simulink model "Mainframe"  (R2021a)
settings: Solver=FixedStepAuto  StartTime=0.0  StopTime=60  FixedStep=0.001  RelTol=1e-3
values from neighbouring files (symbols this model uses):
  den_lpf_d = den_lpf20    [Mainframe_init.m]    (also in load_autopilot.m)
  Emulated_FCC_IO_Delay = 7    [Mainframe_init.m]
  Enable_Gyros = 0    [Mainframe_init.m]
  Enable_INS = 0    [Mainframe_init.m]
  num_lpf_d = num_lpf20    [Mainframe_init.m]    (also in load_autopilot.m)
undefined symbols (not defined in the file or in its folder): act_dmp, act_omega, Actuator, Aerodynamics, aMode, Autopilot, AUX, c_b_WGS, c_be, c_flat, c_grav, c_h_geop0, c_h_geope, c_pa0, c_pe, c_r0, c_rot, c_rsma, c_Tmp0, d_siB_0, d_siB_max, d_siB_min, dd_siB_max, dd_siB_min, dev, DiscIntNeverNeededParam, e_pa, e_Tmp, fin_maxrate, flag_I_act_switch, flag_I_aero_switch, flag_I_flat, flag_I_gravity_switch, flag_I_rot, hcr, HIL_Data, JMMM_0, JMMM_e, JSPB_e, lat_0, lon_0, Mass_Props, mB_0, mM_0, mM_e, National_Instruments, Newton, pBII_0, PCIe, pMPB, pNPB, propellant_kg, prp_FBPB, prp_mdot, prp_T, pSPB, pwm_output1, qEG_0, qIB_0, qIE_0 ... (+31)
libraries: simulink_extras x38, simulink x31, custom_blocks x11, sldrtlib x10, aerolibcommonsys x4, px4Sensorslib x3, px4lib x3, aerolibnav x1
(part 13 of 17)

== system Mainframe/Non-linear Flight Dynamic Model/GRM_Airframe/rb_eom/eom_6dof/Rigid_Body_EOM_6_DOF/rb_eom_6dof/calc_d_qIB ==
  note: Body-Drehraten
      | d_qBI(1) =1/2 { q4wx  - q3wy + q2wz }
      | d_qBI(2) =1/2 { q3wx + q4wy  - q1wz }
      | d_qBI(3) =1/2 {-q2wx + q1wy + q4wz }
      | d_qBI(4) =1/2 {-q1wx  - q2wy  - q3wz }
      |
      | Entspricht Zipfel (s. 372, Gl 10.11)
      | Entspricht "Representing Attitude: Euler angles, Unit Quaternions, and Rotation Vectors",
      | 	J. Diebel, Stanford University, S. 16, Gl 157 oder (159 & 151)
      |
      | d_qBI = 1/2 * [wBIB (1, 2, 3), 0] * qBI
  qIB : Inport
  wBIB : Inport  Port=2
  Add : Sum  Inputs=++++
  Constant : Constant  Value=0
  Demux : Demux  Outputs=3
  Demux1 : Demux
  Gain : Gain  Gain=0.5
  Product{2..5} (4 alike) : Product
  Product6 : Product  Multiplication=Matrix(*)
  Q_1 : Constant  Value=[0 0 0 1; 0 0 1 0; 0 -1 0 0; -1 0 0 0]
  Q_2 : Constant  Value=[0 0 -1 0; 0 0 0 1; 1 0 0 0; 0 -1 0 0]
  Q_3 : Constant  Value=[0 1 0 0; -1 0 0 0; 0 0 0 1; 0 0 -1 0]
  Q_4 : Constant  Value=[1 0 0 0; 0 1 0 0; 0 0 1 0; 0 0 0 1]
  Vector Concatenate : Concatenate  NumInputs=4
  conjugate_quaternion : Subsystem
      mask help: conjugate a quaternion
      mask Help:
      | Name:
      | 
      |     conjugate_quaternion
      | 
      | Description:
      | 
      |     computes the conjugate quaternion
      | 
      | Inputs  [size] [data type] [unit]:
      | 
      |     quaternion q_2_1  [4] [double] [-]
      | 
      | Outputs  [size] [data type] [unit]:
      | 
      |     conjugated quaternion q_1_2  [4] [double] [-]
      mask Display: disp (' conj(q)')
  conjugate_quaternion1 : Subsystem
      mask help: conjugate a quaternion
      mask Help:
      | Name:
      | 
      |     conjugate_quaternion
      | 
      | Description:
      | 
      |     computes the conjugate quaternion
      | 
      | Inputs  [size] [data type] [unit]:
      | 
      |     quaternion q_2_1  [4] [double] [-]
      | 
      | Outputs  [size] [data type] [unit]:
      | 
      |     conjugated quaternion q_1_2  [4] [double] [-]
      mask Display: disp (' conj(q)')
  d_qIB : Outport  VectorParamsAs1DForOutWhenUnconnected=off
  wires:
  conjugate_quaternion1/1(q_conj) -> d_qIB/1  "d_qIB"
  conjugate_quaternion/1(q_conj) -> Product6/2  "qBI"
  Vector Concatenate/1 -> Demux1/1
  Constant/1 -> Vector Concatenate/4
  Demux/3 -> Vector Concatenate/3
  Demux/2 -> Vector Concatenate/2
  Demux/1 -> Vector Concatenate/1
  wBIB/1 -> Demux/1
  qIB/1 -> conjugate_quaternion/1(q)
  Gain/1 -> conjugate_quaternion1/1(q)  "d_qBI"
  Product2/1 -> Add/1
  Product4/1 -> Add/3
  Demux1/4 -> Product5/2  "w4"
  Demux1/3 -> Product4/2  "w3"
  Product3/1 -> Add/2
  Q_2/1 -> Product3/1
  Q_1/1 -> Product2/1
  Demux1/2 -> Product3/2  "w2"
  Q_4/1 -> Product5/1
  Product6/1 -> Gain/1
  Product5/1 -> Add/4
  Demux1/1 -> Product2/2  "w1"
  Add/1 -> Product6/1  "Q(w')"
  Q_3/1 -> Product4/1

== system Mainframe/Non-linear Flight Dynamic Model/GRM_Airframe/rb_eom/eom_6dof/Rigid_Body_EOM_6_DOF/rb_eom_6dof/cross_product ==
  note: Outputs [size]:
      |
      | r1 x r2  [3x1]
  note: Inputs [size]:
      |
      | r1 [3x1]
      | r2 [3x1]
  r1 : Inport
  r2 : Inport  Port=2
  Demux2 : Demux  Outputs=[1;1;1]
      settings: DisplayOption=none
  Demux3 : Demux  Outputs=[1;1;1]
      settings: DisplayOption=none
  Product{2..7} (6 alike) : Product  InputSameDT=on  RndMeth=Zero  SaturateOnIntegerOverflow=on  OutDataTypeStr=Inherit: Same as first input
  Sum : Sum  Inputs=+-  InputSameDT=on  SaturateOnIntegerOverflow=on  OutDataTypeStr=Inherit: Same as first input
  Sum1 : Sum  Inputs=+-  InputSameDT=on  SaturateOnIntegerOverflow=on  OutDataTypeStr=Inherit: Same as first input
  Sum2 : Sum  Inputs=+-  InputSameDT=on  SaturateOnIntegerOverflow=on  OutDataTypeStr=Inherit: Same as first input
  Vector Concatenate : Concatenate  NumInputs=3  Mode=Multidimensional array
  r1_x_r2 : Outport  PortDimensions=[3,1]  VectorParamsAs1DForOutWhenUnconnected=off
  wires:
  Demux2/2 -> Product2/1, Product7/1
  Demux3/3 -> Product5/2, Product2/2
  Demux3/2 -> Product6/2, Product3/2
  Demux2/3 -> Product3/1, Product4/1
  Demux3/1 -> Product7/2, Product4/2
  Demux2/1 -> Product6/1, Product5/1
  Product2/1 -> Sum/1
  Product3/1 -> Sum/2
  Product4/1 -> Sum1/1
  Product5/1 -> Sum1/2
  Product6/1 -> Sum2/1
  Product7/1 -> Sum2/2
  Sum/1 -> Vector Concatenate/1
  Sum1/1 -> Vector Concatenate/2
  Sum2/1 -> Vector Concatenate/3
  r1/1 -> Demux2/1
  r2/1 -> Demux3/1
  Vector Concatenate/1 -> r1_x_r2/1

== system Mainframe/Non-linear Flight Dynamic Model/GRM_Airframe/rb_eom/eom_6dof/Rigid_Body_EOM_6_DOF/rb_eom_6dof/r2_from_r1_trans_q21 ==
  note: Outputs [size]:
      |
      | vector r2 [3]
  note: Inputs [size]:
      |
      | vector r1 [3]
      | quaternion q21 [4]
  r1 : Inport
  q21 : Inport  Port=2
  Add : Sum  Inputs=++++
  Add1 : Sum  Inputs=++++
  Constant : Constant  Value=0
  Demux : Demux  Outputs=3
  Demux1 : Demux
  Demux2 : Demux
  Math Function : Math  Operator=transpose  SignedPower=on  SaturateOnIntegerOverflow=on
  Product{,1..7} (8 alike) : Product
  Product8 : Product  Inputs=3  Multiplication=Matrix(*)
  Q_1 : Constant  Value=[0 0 0 1; 0 0 1 0; 0 -1 0 0; -1 0 0 0]
  Q_2 : Constant  Value=[0 0 -1 0; 0 0 0 1; 1 0 0 0; 0 -1 0 0]
  Q_3 : Constant  Value=[0 1 0 0; -1 0 0 0; 0 0 0 1; 0 0 -1 0]
  Q_4 : Constant  Value=[1 0 0 0; 0 1 0 0; 0 0 1 0; 0 0 0 1]
  Q~_1 : Constant  Value=[0 0 0 1; 0 0 -1 0; 0 1 0 0; -1 0 0 0]
  Q~_2 : Constant  Value=[0 0 1 0; 0 0 0 1; -1 0 0 0; 0 -1 0 0]
  Q~_3 : Constant  Value=[0 -1 0 0; 1 0 0 0; 0 0 0 1; 0 0 -1 0]
  Q~_4 : Constant  Value=[1 0 0 0; 0 1 0 0; 0 0 1 0; 0 0 0 1]
  Selector : Selector  IndexMode=Zero-based  InputPortWidth=4  IndexOptions=Index vector (dialog)  Indices=[0 1 2]  OutputSizes=1
  Vector Concatenate : Concatenate  NumInputs=4
  r2 : Outport  VectorParamsAs1DForOutWhenUnconnected=off
  wires:
  Selector/1 -> r2/1
  Product8/1 -> Selector/1
  Vector Concatenate/1 -> Product8/3
  Constant/1 -> Vector Concatenate/4
  Math Function/1 -> Product8/1  "Q~T(q)"
  Q~_3/1 -> Product6/1
  Q~_1/1 -> Product4/1
  Q~_4/1 -> Product7/1
  Product6/1 -> Add1/3
  Demux2/3 -> Product6/2  "q3"
  Product5/1 -> Add1/2
  Demux2/2 -> Product5/2  "q2"
  Add1/1 -> Math Function/1  "Q~(q)"
  q21/1 -> Demux1/1, Demux2/1
  Product7/1 -> Add1/4
  Product4/1 -> Add1/1
  Q~_2/1 -> Product5/1
  Demux2/4 -> Product7/2  "q4"
  Demux2/1 -> Product4/2  "q1"
  Add/1 -> Product8/2  "Q(q)"
  Product3/1 -> Add/4
  Product2/1 -> Add/3
  Product1/1 -> Add/2
  Product/1 -> Add/1
  Q_4/1 -> Product3/1
  Q_3/1 -> Product2/1
  Q_2/1 -> Product1/1
  Q_1/1 -> Product/1
  Demux1/4 -> Product3/2  "q4"
  Demux1/3 -> Product2/2  "q3"
  Demux1/2 -> Product1/2  "q2"
  Demux1/1 -> Product/2  "q1"
  Demux/3 -> Vector Concatenate/3  "rz"
  Demux/2 -> Vector Concatenate/2  "ry"
  Demux/1 -> Vector Concatenate/1  "rx"
  r1/1 -> Demux/1

== system Mainframe/Non-linear Flight Dynamic Model/GRM_Airframe/stream_flow/calc_stream_flow/Subsystem1/AoA_Sideslip_Alphatot_Phi/norm_of_vector ==
  note: Outputs [size]:
      |
      | norm of vector [1]
  note: Inputs [size]:
      |
      | vector  [3]
  vector : Inport
  Dot Product1 : DotProduct  InputSameDT=on  OutDataTypeStr=Inherit: Inherit via internal rule
  Math Function1 : Math  Operator=sqrt  SignedPower=on  SaturateOnIntegerOverflow=on
  norm_of_vector : Outport  VectorParamsAs1DForOutWhenUnconnected=off
  wires:
  vector/1 -> Dot Product1/1, Dot Product1/2
  Math Function1/1 -> norm_of_vector/1
  Dot Product1/1 -> Math Function1/1

== system Mainframe/Non-linear Flight Dynamic Model/GRM_Airframe/weight_and_balance/moi/moi_coordinate_transformation/3_rot_mat/1. Rotation x-Achse ==
  alpha1 : Inport
  Constant : Constant
  Constant{1..2,7..8} (4 alike) : Constant  Value=0
  Gain : Gain  Gain=-1
  Matrix Concatenate : Concatenate  NumInputs=3  Mode=Multidimensional array  ConcatenateDimension=2
  Mux : Mux  Inputs=3
  Mux1 : Mux  Inputs=3
  Mux2 : Mux  Inputs=3
  Trigonometric Function : Trigonometry  Operator=cos
  Trigonometric Function1 : Trigonometry
  Trigonometric Function2 : Trigonometry
  Trigonometric Function3 : Trigonometry  Operator=cos
  1Rot_Matrix_x : Outport  VectorParamsAs1DForOutWhenUnconnected=off
  wires:
  Gain/1 -> Mux1/3
  alpha1/1 -> Trigonometric Function2/1, Trigonometric Function/1, Trigonometric Function1/1, Trigonometric Function3/1
  Constant/1 -> Mux/1
  Constant1/1 -> Mux/2
  Constant2/1 -> Mux/3
  Constant8/1 -> Mux1/1
  Trigonometric Function/1 -> Mux1/2
  Trigonometric Function2/1 -> Gain/1
  Constant7/1 -> Mux2/1
  Trigonometric Function1/1 -> Mux2/2
  Trigonometric Function3/1 -> Mux2/3
  Mux/1 -> Matrix Concatenate/1
  Mux1/1 -> Matrix Concatenate/2
  Mux2/1 -> Matrix Concatenate/3
  Matrix Concatenate/1 -> 1Rot_Matrix_x/1

== system Mainframe/Non-linear Flight Dynamic Model/GRM_Airframe/weight_and_balance/moi/moi_coordinate_transformation/3_rot_mat/1. Rotation y-Achse ==
  alpha1 : Inport
  Constant{,2,7..8} (4 alike) : Constant  Value=0
  Constant1 : Constant
  Gain1 : Gain  Gain=-1
  Matrix Concatenate : Concatenate  NumInputs=3  Mode=Multidimensional array  ConcatenateDimension=2
  Mux : Mux  Inputs=3
  Mux1 : Mux  Inputs=3
  Mux2 : Mux  Inputs=3
  Trigonometric Function : Trigonometry  Operator=cos
  Trigonometric Function1 : Trigonometry
  Trigonometric Function2 : Trigonometry
  Trigonometric Function3 : Trigonometry  Operator=cos
  1Rot_Matrix_y : Outport  VectorParamsAs1DForOutWhenUnconnected=off
  wires:
  Gain1/1 -> Mux2/1
  Mux2/1 -> Matrix Concatenate/3
  Mux1/1 -> Matrix Concatenate/2
  Mux/1 -> Matrix Concatenate/1
  Trigonometric Function3/1 -> Mux2/3
  Trigonometric Function1/1 -> Gain1/1
  Constant2/1 -> Mux1/3
  Constant1/1 -> Mux1/2
  Constant/1 -> Mux1/1
  alpha1/1 -> Trigonometric Function1/1, Trigonometric Function3/1, Trigonometric Function2/1, Trigonometric Function/1
  Constant8/1 -> Mux/2
  Trigonometric Function/1 -> Mux/1
  Trigonometric Function2/1 -> Mux/3
  Constant7/1 -> Mux2/2
  Matrix Concatenate/1 -> 1Rot_Matrix_y/1

== system Mainframe/Non-linear Flight Dynamic Model/GRM_Airframe/weight_and_balance/moi/moi_coordinate_transformation/3_rot_mat/1. Rotation z-Achse ==
  alpha1 : Inport
  Constant{4,7..8,10} (4 alike) : Constant  Value=0
  Constant11 : Constant
  Gain : Gain  Gain=-1
  Matrix Concatenate : Concatenate  NumInputs=3  Mode=Multidimensional array  ConcatenateDimension=2
  Mux : Mux  Inputs=3
  Mux1 : Mux  Inputs=3
  Mux2 : Mux  Inputs=3
  Trigonometric Function : Trigonometry  Operator=cos
  Trigonometric Function1 : Trigonometry
  Trigonometric Function3 : Trigonometry  Operator=cos
  Trigonometric Function4 : Trigonometry
  1Rot_Matrix_z : Outport  VectorParamsAs1DForOutWhenUnconnected=off
  wires:
  Gain/1 -> Mux/2
  Trigonometric Function/1 -> Mux1/2
  Mux/1 -> Matrix Concatenate/1
  Mux1/1 -> Matrix Concatenate/2
  Mux2/1 -> Matrix Concatenate/3
  Trigonometric Function1/1 -> Mux1/1
  Constant7/1 -> Mux1/3
  Constant4/1 -> Mux2/1
  Constant10/1 -> Mux2/2
  Constant11/1 -> Mux2/3
  Trigonometric Function3/1 -> Mux/1
  Trigonometric Function4/1 -> Gain/1
  Constant8/1 -> Mux/3
  Matrix Concatenate/1 -> 1Rot_Matrix_z/1
  alpha1/1 -> Trigonometric Function3/1, Trigonometric Function4/1, Trigonometric Function/1, Trigonometric Function1/1

== system Mainframe/Non-linear Flight Dynamic Model/GRM_Airframe/weight_and_balance/moi/moi_coordinate_transformation/3_rot_mat/2. Rotation x-Achse ==
  alpha2 : Inport
  Constant : Constant
  Constant{1..2,7..8} (4 alike) : Constant  Value=0
  Gain : Gain  Gain=-1
  Matrix Concatenate : Concatenate  NumInputs=3  Mode=Multidimensional array  ConcatenateDimension=2
  Mux : Mux  Inputs=3
  Mux1 : Mux  Inputs=3
  Mux2 : Mux  Inputs=3
  Trigonometric Function : Trigonometry  Operator=cos
  Trigonometric Function1 : Trigonometry
  Trigonometric Function2 : Trigonometry
  Trigonometric Function3 : Trigonometry  Operator=cos
  2Rot_Matrix_x : Outport  VectorParamsAs1DForOutWhenUnconnected=off
  wires:
  Gain/1 -> Mux1/3
  alpha2/1 -> Trigonometric Function2/1, Trigonometric Function/1, Trigonometric Function1/1, Trigonometric Function3/1
  Constant/1 -> Mux/1
  Constant1/1 -> Mux/2
  Constant2/1 -> Mux/3
  Constant8/1 -> Mux1/1
  Trigonometric Function/1 -> Mux1/2
  Trigonometric Function2/1 -> Gain/1
  Constant7/1 -> Mux2/1
  Trigonometric Function1/1 -> Mux2/2
  Trigonometric Function3/1 -> Mux2/3
  Mux/1 -> Matrix Concatenate/1
  Mux1/1 -> Matrix Concatenate/2
  Mux2/1 -> Matrix Concatenate/3
  Matrix Concatenate/1 -> 2Rot_Matrix_x/1

== system Mainframe/Non-linear Flight Dynamic Model/GRM_Airframe/weight_and_balance/moi/moi_coordinate_transformation/3_rot_mat/2. Rotation y-Achse ==
  alpha2 : Inport
  Constant{,2,7..8} (4 alike) : Constant  Value=0
  Constant1 : Constant
  Gain1 : Gain  Gain=-1
  Matrix Concatenate : Concatenate  NumInputs=3  Mode=Multidimensional array  ConcatenateDimension=2
  Mux : Mux  Inputs=3
  Mux1 : Mux  Inputs=3
  Mux2 : Mux  Inputs=3
  Trigonometric Function : Trigonometry  Operator=cos
  Trigonometric Function1 : Trigonometry
  Trigonometric Function2 : Trigonometry
  Trigonometric Function3 : Trigonometry  Operator=cos
  2Rot_Matrix_y : Outport  VectorParamsAs1DForOutWhenUnconnected=off
  wires:
  Gain1/1 -> Mux2/1
  Mux2/1 -> Matrix Concatenate/3
  Mux1/1 -> Matrix Concatenate/2
  Mux/1 -> Matrix Concatenate/1
  Trigonometric Function3/1 -> Mux2/3
  Trigonometric Function1/1 -> Gain1/1
  Constant2/1 -> Mux1/3
  Constant1/1 -> Mux1/2
  Constant/1 -> Mux1/1
  alpha2/1 -> Trigonometric Function1/1, Trigonometric Function3/1, Trigonometric Function2/1, Trigonometric Function/1
  Constant8/1 -> Mux/2
  Trigonometric Function/1 -> Mux/1
  Trigonometric Function2/1 -> Mux/3
  Constant7/1 -> Mux2/2
  Matrix Concatenate/1 -> 2Rot_Matrix_y/1

== system Mainframe/Non-linear Flight Dynamic Model/GRM_Airframe/weight_and_balance/moi/moi_coordinate_transformation/3_rot_mat/2. Rotation z-Achse ==
  alpha2 : Inport
  Constant{4,7..8,10} (4 alike) : Constant  Value=0
  Constant11 : Constant
  Gain : Gain  Gain=-1
  Matrix Concatenate : Concatenate  NumInputs=3  Mode=Multidimensional array  ConcatenateDimension=2
  Mux : Mux  Inputs=3
  Mux1 : Mux  Inputs=3
  Mux2 : Mux  Inputs=3
  Trigonometric Function : Trigonometry  Operator=cos
  Trigonometric Function1 : Trigonometry
  Trigonometric Function3 : Trigonometry  Operator=cos
  Trigonometric Function4 : Trigonometry
  2Rot_Matrix_z : Outport  VectorParamsAs1DForOutWhenUnconnected=off
  wires:
  Gain/1 -> Mux/2
  Trigonometric Function/1 -> Mux1/2
  Mux/1 -> Matrix Concatenate/1
  Mux1/1 -> Matrix Concatenate/2
  Mux2/1 -> Matrix Concatenate/3
  Trigonometric Function1/1 -> Mux1/1
  Constant7/1 -> Mux1/3
  Constant4/1 -> Mux2/1
  Constant10/1 -> Mux2/2
  Constant11/1 -> Mux2/3
  Trigonometric Function3/1 -> Mux/1
  Trigonometric Function4/1 -> Gain/1
  Constant8/1 -> Mux/3
  Matrix Concatenate/1 -> 2Rot_Matrix_z/1
  alpha2/1 -> Trigonometric Function3/1, Trigonometric Function4/1, Trigonometric Function/1, Trigonometric Function1/1

== system Mainframe/Non-linear Flight Dynamic Model/GRM_Airframe/weight_and_balance/moi/moi_coordinate_transformation/3_rot_mat/3. Rotation x-Achse ==
  alpha3 : Inport
  Constant : Constant
  Constant{1..2,7..8} (4 alike) : Constant  Value=0
  Gain : Gain  Gain=-1
  Matrix Concatenate : Concatenate  NumInputs=3  Mode=Multidimensional array  ConcatenateDimension=2
  Mux : Mux  Inputs=3
  Mux1 : Mux  Inputs=3
  Mux2 : Mux  Inputs=3
  Trigonometric Function : Trigonometry  Operator=cos
  Trigonometric Function1 : Trigonometry
  Trigonometric Function2 : Trigonometry
  Trigonometric Function3 : Trigonometry  Operator=cos
  3Rot_Matrix_x : Outport  VectorParamsAs1DForOutWhenUnconnected=off
  wires:
  Gain/1 -> Mux1/3
  alpha3/1 -> Trigonometric Function2/1, Trigonometric Function/1, Trigonometric Function1/1, Trigonometric Function3/1
  Constant/1 -> Mux/1
  Constant1/1 -> Mux/2
  Constant2/1 -> Mux/3
  Constant8/1 -> Mux1/1
  Trigonometric Function/1 -> Mux1/2
  Trigonometric Function2/1 -> Gain/1
  Constant7/1 -> Mux2/1
  Trigonometric Function1/1 -> Mux2/2
  Trigonometric Function3/1 -> Mux2/3
  Mux/1 -> Matrix Concatenate/1
  Mux1/1 -> Matrix Concatenate/2
  Mux2/1 -> Matrix Concatenate/3
  Matrix Concatenate/1 -> 3Rot_Matrix_x/1

== system Mainframe/Non-linear Flight Dynamic Model/GRM_Airframe/weight_and_balance/moi/moi_coordinate_transformation/3_rot_mat/3. Rotation y-Achse ==
  alpha3 : Inport
  Constant{,2,7..8} (4 alike) : Constant  Value=0
  Constant1 : Constant
  Gain1 : Gain  Gain=-1
  Matrix Concatenate : Concatenate  NumInputs=3  Mode=Multidimensional array  ConcatenateDimension=2
  Mux : Mux  Inputs=3
  Mux1 : Mux  Inputs=3
  Mux2 : Mux  Inputs=3
  Trigonometric Function : Trigonometry  Operator=cos
  Trigonometric Function1 : Trigonometry
  Trigonometric Function2 : Trigonometry
  Trigonometric Function3 : Trigonometry  Operator=cos
  3Rot_Matrix_y : Outport  VectorParamsAs1DForOutWhenUnconnected=off
  wires:
  Gain1/1 -> Mux2/1
  Mux2/1 -> Matrix Concatenate/3
  Mux1/1 -> Matrix Concatenate/2
  Mux/1 -> Matrix Concatenate/1
  Trigonometric Function3/1 -> Mux2/3
  Trigonometric Function1/1 -> Gain1/1
  Constant2/1 -> Mux1/3
  Constant1/1 -> Mux1/2
  Constant/1 -> Mux1/1
  alpha3/1 -> Trigonometric Function1/1, Trigonometric Function3/1, Trigonometric Function2/1, Trigonometric Function/1
  Constant8/1 -> Mux/2
  Trigonometric Function/1 -> Mux/1
  Trigonometric Function2/1 -> Mux/3
  Constant7/1 -> Mux2/2
  Matrix Concatenate/1 -> 3Rot_Matrix_y/1

== system Mainframe/Non-linear Flight Dynamic Model/GRM_Airframe/weight_and_balance/moi/moi_coordinate_transformation/3_rot_mat/3. Rotation z-Achse ==
  alpha3 : Inport
  Constant{4,7..8,10} (4 alike) : Constant  Value=0
  Constant11 : Constant
  Gain : Gain  Gain=-1
  Matrix Concatenate : Concatenate  NumInputs=3  Mode=Multidimensional array  ConcatenateDimension=2
  Mux : Mux  Inputs=3
  Mux1 : Mux  Inputs=3
  Mux2 : Mux  Inputs=3
  Trigonometric Function : Trigonometry  Operator=cos
  Trigonometric Function1 : Trigonometry
  Trigonometric Function3 : Trigonometry  Operator=cos
  Trigonometric Function4 : Trigonometry
  3Rot_Matrix_z : Outport  VectorParamsAs1DForOutWhenUnconnected=off
  wires:
  Gain/1 -> Mux/2
  Trigonometric Function/1 -> Mux1/2
  Mux/1 -> Matrix Concatenate/1
  Mux1/1 -> Matrix Concatenate/2
  Mux2/1 -> Matrix Concatenate/3
  Trigonometric Function1/1 -> Mux1/1
  Constant7/1 -> Mux1/3
  Constant4/1 -> Mux2/1
  Constant10/1 -> Mux2/2
  Constant11/1 -> Mux2/3
  Trigonometric Function3/1 -> Mux/1
  Trigonometric Function4/1 -> Gain/1
  Constant8/1 -> Mux/3
  Matrix Concatenate/1 -> 3Rot_Matrix_z/1
  alpha3/1 -> Trigonometric Function3/1, Trigonometric Function4/1, Trigonometric Function/1, Trigonometric Function1/1

== system Mainframe/Non-linear Flight Dynamic Model/Subsystem1/Extract States/Assemble_States_Bus1/Three-axis Inertial Measurement Unit3/Three-axis Accelerometer/Dynamics ==
  sp_f : Inport
  Constant : Constant  Value=dtype_a
  No Dynamics : Subsystem
  Second-order Dynamics : Subsystem  mask(ContinuousFilter){wn=w_a, zn=z_a}
      mask prompts: wn "Natural frequency:"; zn "Damping ratio:"
      mask init:
      | aeroicon('aeroblk');
  Switch : Switch  Threshold=0.5
  "sp_f " : Outport  VectorParamsAs1DForOutWhenUnconnected=off
  wires:
  Constant/1 -> Switch/2
  Switch/1 -> "sp_f "/1
  Second-order Dynamics/1(Out) -> Switch/1
  No Dynamics/1(Out1) -> Switch/3
  sp_f/1 -> Second-order Dynamics/1(In), No Dynamics/1(In1)

== system Mainframe/Non-linear Flight Dynamic Model/Subsystem1/Extract States/Assemble_States_Bus1/Three-axis Inertial Measurement Unit3/Three-axis Accelerometer/w x (w x d) ==
  "p q r " : Inport
  distance : Inport  Port=2
  w x (w x d) : Subsystem  mask(CrossProduct){aMode=aMode}
      mask help: shared_aeroblks:sharedaeroblkutil:blockCrossProductDesc
      mask init:
      | if aerosharedtest(gcb)
      |     aerosharedicon('shared');
      | else
      |     sharedautoicon('shared');
      | end
      mask Help: eval('if license(''test'',''Aerospace_Blockset'')aerosharedhelp(''threebythree_cross_product'');elseif license(''test'',''Powertrain_Blockset'')sharedautohelp(''threebythree_cross_product'');end')
      mask Display:
      | text(.5,.5,'Cross\nProduct\nC = AxB', ...
      | 	'HorizontalAlignment','Center',...
      | 	'VerticalAlignment','middle')
  w x d : Subsystem  mask(CrossProduct){aMode=aMode}
      mask help: shared_aeroblks:sharedaeroblkutil:blockCrossProductDesc
      mask init:
      | if aerosharedtest(gcb)
      |     aerosharedicon('shared');
      | else
      |     sharedautoicon('shared');
      | end
      mask Help: eval('if license(''test'',''Aerospace_Blockset'')aerosharedhelp(''threebythree_cross_product'');elseif license(''test'',''Powertrain_Blockset'')sharedautohelp(''threebythree_cross_product'');end')
      mask Display:
      | text(.5,.5,'Cross\nProduct\nC = AxB', ...
      | 	'HorizontalAlignment','Center',...
      | 	'VerticalAlignment','middle')
  w x ( w x d) : Outport  VectorParamsAs1DForOutWhenUnconnected=off
  wires:
  "p q r "/1 -> w x (w x d)/1(A), w x d/1(A)
  w x d/1(C) -> w x (w x d)/2(B)
  distance/1 -> w x d/2(B)
  w x (w x d)/1(C) -> w x ( w x d)/1

== system Mainframe/Non-linear Flight Dynamic Model/Subsystem1/Extract States/Assemble_States_Bus1/Three-axis Inertial Measurement Unit3/Three-axis Accelerometer/wdot x d ==
  A : Inport
  B : Inport  Port=2
  "A " : InportShadow
  "B " : InportShadow  Port=2
  Subsystem : Subsystem
  Subsystem1 : Subsystem
  Sum : Sum  Inputs=+|-  InputSameDT=on  SaturateOnIntegerOverflow=on  OutDataTypeStr=Inherit: Same as first input
  C : Outport  VectorParamsAs1DForOutWhenUnconnected=off
  wires:
  Subsystem1/1(Out1) -> Sum/2
  Subsystem/1(Out1) -> Sum/1
  A/1 -> Subsystem/1(A)
  B/1 -> Subsystem/2(B)
  Sum/1 -> C/1
  "A "/1 -> Subsystem1/1(A)
  "B "/1 -> Subsystem1/2(B)

== system Mainframe/Non-linear Flight Dynamic Model/Subsystem1/Extract States/Assemble_States_Bus1/Three-axis Inertial Measurement Unit3/Three-axis Gyroscope/Dynamics ==
  p q r : Inport
  Constant : Constant  Value=dtype_g
  No Dynamics : Subsystem
  Second-order Dynamics : Subsystem  mask(ContinuousFilter){wn=w_g, zn=z_g}
      mask prompts: wn "Natural frequency:"; zn "Damping ratio:"
      mask init:
      | aeroicon('aeroblk');
  Switch : Switch  Threshold=0.5
  "p q r " : Outport  VectorParamsAs1DForOutWhenUnconnected=off
  wires:
  p q r/1 -> Second-order Dynamics/1(In), No Dynamics/1(In1)
  No Dynamics/1(Out1) -> Switch/3
  Second-order Dynamics/1(Out) -> Switch/1
  Switch/1 -> "p q r "/1
  Constant/1 -> Switch/2

== system Mainframe/Non-linear Flight Dynamic Model/Subsystem1/GRM_Airframe/aerodynamics/aerodynamic_via_lookup/calc_aero_coefficients/CLL_TLU ==
  alpha_deg : Inport
  beta_deg : Inport  Port=2
  dele_deg : Inport  Port=3
  dela_deg : Inport  Port=4
  delr_deg : Inport  Port=5
  p_ND_rps : Inport  Port=6
  1-D Lookup Table : Lookup_n-D  NumberOfTableDimensions=1  BreakpointsForDimension1=Aerodynamics.alpha_bkpts_ind1  Table=Aerodynamics.CLL_alpha  ExtrapMethod=Clip  UseLastTableValue=on  InternalRulePriority=Speed  RndMeth=Simplest  InputSameDT=on
      settings: AttributesFormatString=|
      | %<Table>
      | %<BreakpointsForDimension1>
  1-D Lookup Table1 : Lookup_n-D  NumberOfTableDimensions=1  BreakpointsForDimension1=Aerodynamics.beta_bkpts_ind1  Table=Aerodynamics.CLL_beta  ExtrapMethod=Clip  UseLastTableValue=on  InternalRulePriority=Speed  RndMeth=Simplest  InputSameDT=on
      settings: AttributesFormatString=|
      | %<Table>
      | %<BreakpointsForDimension1>
  2-D Lookup Table : Lookup_n-D  BreakpointsForDimension1=Aerodynamics.dele_inc_bkpts_ind1  BreakpointsForDimension2=Aerodynamics.dele_inc_bkpts_ind2  Table=Aerodynamics.CLL_dele_inc  ExtrapMethod=Clip  UseLastTableValue=on  InternalRulePriority=Speed  RndMeth=Simplest  InputSameDT=on
      settings: InputPortMap=u0,u1
      settings: AttributesFormatString=|
      | %<Table>
      | %<BreakpointsForDimension1>
      | %<BreakpointsForDimension2>
  2-D Lookup Table1 : Lookup_n-D  BreakpointsForDimension1=Aerodynamics.dela_inc_bkpts_ind1  BreakpointsForDimension2=Aerodynamics.dela_inc_bkpts_ind2  Table=Aerodynamics.CLL_dela_inc  ExtrapMethod=Clip  UseLastTableValue=on  InternalRulePriority=Speed  RndMeth=Simplest  InputSameDT=on
      settings: InputPortMap=u0,u1
      settings: AttributesFormatString=|
      | %<Table>
      | %<BreakpointsForDimension1>
      | %<BreakpointsForDimension2>
  2-D Lookup Table2 : Lookup_n-D  BreakpointsForDimension1=Aerodynamics.delr_inc_bkpts_ind1  BreakpointsForDimension2=Aerodynamics.delr_inc_bkpts_ind2  Table=Aerodynamics.CLL_delr_inc  ExtrapMethod=Clip  UseLastTableValue=on  InternalRulePriority=Speed  RndMeth=Simplest  InputSameDT=on
      settings: InputPortMap=u0,u1
      settings: AttributesFormatString=|
      | %<Table>
      | %<BreakpointsForDimension1>
      | %<BreakpointsForDimension2>
  Constant : Constant  Value=Aerodynamics.CLL_bias
      settings: AttributesFormatString=%<Value>
  Gain : Gain  Gain=Aerodynamics.CLL_scale
      settings: AttributesFormatString=%<Gain>
  Gain2 : Gain  Gain=Aerodynamics.CLL_p
      settings: AttributesFormatString=%<Gain>
  Sum1 : Sum  Inputs=+++++
  Sum2 : Sum
  Sum3 : Sum  Inputs=|++
  alpha_deg D1 : InportShadow
  alpha_deg D2 : InportShadow
  beta_deg D1 : InportShadow  Port=2
  CLL : Outport
  wires:
  p_ND_rps/1 -> Gain2/1
  Gain2/1 -> Sum1/5
  Gain/1 -> Sum3/1
  2-D Lookup Table2/1 -> Sum1/4  "CLL_delr"
  1-D Lookup Table/1 -> Sum2/1
  2-D Lookup Table1/1 -> Sum1/3  "CLL_dela"
  beta_deg/1 -> 1-D Lookup Table1/1
  1-D Lookup Table1/1 -> Sum2/2
  2-D Lookup Table/1 -> Sum1/2  "CLL_dele"
  dele_deg/1 -> 2-D Lookup Table/2
  alpha_deg D1/1 -> 2-D Lookup Table/1
  beta_deg D1/1 -> 2-D Lookup Table2/1
  dela_deg/1 -> 2-D Lookup Table1/2
  alpha_deg/1 -> 1-D Lookup Table/1
  alpha_deg D2/1 -> 2-D Lookup Table1/1
  delr_deg/1 -> 2-D Lookup Table2/2
  Sum2/1 -> Sum1/1  "CLL_0"
  Constant/1 -> Sum3/2
  Sum1/1 -> Gain/1
  Sum3/1 -> CLL/1  "CLL_B"

== system Mainframe/Non-linear Flight Dynamic Model/Subsystem1/GRM_Airframe/aerodynamics/aerodynamic_via_lookup/calc_aero_coefficients/CLM_TLU ==
  alpha_deg : Inport
  beta_deg : Inport  Port=2
  dele_deg : Inport  Port=3
  dela_deg : Inport  Port=4
  delr_deg : Inport  Port=5
  q_ND_rps : Inport  Port=6
  1-D Lookup Table : Lookup_n-D  NumberOfTableDimensions=1  BreakpointsForDimension1=Aerodynamics.alpha_bkpts_ind1  Table=Aerodynamics.CLM_alpha  ExtrapMethod=Clip  UseLastTableValue=on  InternalRulePriority=Speed  RndMeth=Simplest  InputSameDT=on
      settings: AttributesFormatString=|
      | %<Table>
      | %<BreakpointsForDimension1>
  1-D Lookup Table1 : Lookup_n-D  NumberOfTableDimensions=1  BreakpointsForDimension1=Aerodynamics.beta_bkpts_ind1  Table=Aerodynamics.CLM_beta  ExtrapMethod=Clip  UseLastTableValue=on  InternalRulePriority=Speed  RndMeth=Simplest  InputSameDT=on
      settings: AttributesFormatString=|
      | %<Table>
      | %<BreakpointsForDimension1>
  2-D Lookup Table : Lookup_n-D  BreakpointsForDimension1=Aerodynamics.dele_inc_bkpts_ind1  BreakpointsForDimension2=Aerodynamics.dele_inc_bkpts_ind2  Table=Aerodynamics.CLM_dele_inc  ExtrapMethod=Clip  UseLastTableValue=on  InternalRulePriority=Speed  RndMeth=Simplest  InputSameDT=on
      settings: InputPortMap=u0,u1
      settings: AttributesFormatString=|
      | %<Table>
      | %<BreakpointsForDimension1>
      | %<BreakpointsForDimension2>
  2-D Lookup Table1 : Lookup_n-D  BreakpointsForDimension1=Aerodynamics.dela_inc_bkpts_ind1  BreakpointsForDimension2=Aerodynamics.dela_inc_bkpts_ind2  Table=Aerodynamics.CLM_dela_inc  ExtrapMethod=Clip  UseLastTableValue=on  InternalRulePriority=Speed  RndMeth=Simplest  InputSameDT=on
      settings: InputPortMap=u0,u1
      settings: AttributesFormatString=|
      | %<Table>
      | %<BreakpointsForDimension1>
      | %<BreakpointsForDimension2>
  2-D Lookup Table2 : Lookup_n-D  BreakpointsForDimension1=Aerodynamics.delr_inc_bkpts_ind1  BreakpointsForDimension2=Aerodynamics.delr_inc_bkpts_ind2  Table=Aerodynamics.CLM_delr_inc  ExtrapMethod=Clip  UseLastTableValue=on  InternalRulePriority=Speed  RndMeth=Simplest  InputSameDT=on
      settings: InputPortMap=u0,u1
      settings: AttributesFormatString=|
      | %<Table>
      | %<BreakpointsForDimension1>
      | %<BreakpointsForDimension2>
  Constant : Constant  Value=Aerodynamics.CLM_bias
      settings: AttributesFormatString=%<Value>
  Gain : Gain  Gain=Aerodynamics.CLM_scale
      settings: AttributesFormatString=%<Gain>
  Gain2 : Gain  Gain=Aerodynamics.CLM_q
      settings: AttributesFormatString=%<Gain>
  Sum1 : Sum  Inputs=+++++
  Sum2 : Sum
  Sum3 : Sum  Inputs=|++
  alpha_deg D1 : InportShadow
  alpha_deg D2 : InportShadow
  beta_deg D1 : InportShadow  Port=2
  CLM : Outport
  wires:
  q_ND_rps/1 -> Gain2/1
  Gain2/1 -> Sum1/5
  Sum3/1 -> CLM/1  "CLM_B"
  delr_deg/1 -> 2-D Lookup Table2/2
  alpha_deg D2/1 -> 2-D Lookup Table1/1
  dela_deg/1 -> 2-D Lookup Table1/2
  alpha_deg/1 -> 1-D Lookup Table/1
  beta_deg D1/1 -> 2-D Lookup Table2/1
  alpha_deg D1/1 -> 2-D Lookup Table/1
  1-D Lookup Table1/1 -> Sum2/2
  dele_deg/1 -> 2-D Lookup Table/2
  2-D Lookup Table/1 -> Sum1/2  "CLM_dele"
  2-D Lookup Table1/1 -> Sum1/3  "CLM_dela"
  beta_deg/1 -> 1-D Lookup Table1/1
  2-D Lookup Table2/1 -> Sum1/4  "CLM_delr"
  Sum2/1 -> Sum1/1  "CLM_0"
  1-D Lookup Table/1 -> Sum2/1
  Sum1/1 -> Gain/1
  Constant/1 -> Sum3/2
  Gain/1 -> Sum3/1

== system Mainframe/Non-linear Flight Dynamic Model/Subsystem1/GRM_Airframe/aerodynamics/aerodynamic_via_lookup/calc_aero_coefficients/CLN_TLU ==
  alpha_deg : Inport
  beta_deg : Inport  Port=2
  dele_deg : Inport  Port=3
  dela_deg : Inport  Port=4
  delr_deg : Inport  Port=5
  r_ND_rps : Inport  Port=6
  1-D Lookup Table : Lookup_n-D  NumberOfTableDimensions=1  BreakpointsForDimension1=Aerodynamics.alpha_bkpts_ind1  Table=Aerodynamics.CLN_alpha  ExtrapMethod=Clip  UseLastTableValue=on  InternalRulePriority=Speed  RndMeth=Simplest  InputSameDT=on
      settings: AttributesFormatString=|
      | %<Table>
      | %<BreakpointsForDimension1>
  1-D Lookup Table1 : Lookup_n-D  NumberOfTableDimensions=1  BreakpointsForDimension1=Aerodynamics.beta_bkpts_ind1  Table=Aerodynamics.CLN_beta  ExtrapMethod=Clip  UseLastTableValue=on  InternalRulePriority=Speed  RndMeth=Simplest  InputSameDT=on
      settings: AttributesFormatString=|
      | %<Table>
      | %<BreakpointsForDimension1>
  2-D Lookup Table : Lookup_n-D  BreakpointsForDimension1=Aerodynamics.dele_inc_bkpts_ind1  BreakpointsForDimension2=Aerodynamics.dele_inc_bkpts_ind2  Table=Aerodynamics.CLN_dele_inc  ExtrapMethod=Clip  UseLastTableValue=on  InternalRulePriority=Speed  RndMeth=Simplest  InputSameDT=on
      settings: InputPortMap=u0,u1
      settings: AttributesFormatString=|
      | %<Table>
      | %<BreakpointsForDimension1>
      | %<BreakpointsForDimension2>
  2-D Lookup Table1 : Lookup_n-D  BreakpointsForDimension1=Aerodynamics.dela_inc_bkpts_ind1  BreakpointsForDimension2=Aerodynamics.dela_inc_bkpts_ind2  Table=Aerodynamics.CLN_dela_inc  ExtrapMethod=Clip  UseLastTableValue=on  InternalRulePriority=Speed  RndMeth=Simplest  InputSameDT=on
      settings: InputPortMap=u0,u1
      settings: AttributesFormatString=|
      | %<Table>
      | %<BreakpointsForDimension1>
      | %<BreakpointsForDimension2>
  2-D Lookup Table2 : Lookup_n-D  BreakpointsForDimension1=Aerodynamics.delr_inc_bkpts_ind1  BreakpointsForDimension2=Aerodynamics.delr_inc_bkpts_ind2  Table=Aerodynamics.CLN_delr_inc  ExtrapMethod=Clip  UseLastTableValue=on  InternalRulePriority=Speed  RndMeth=Simplest  InputSameDT=on
      settings: InputPortMap=u0,u1
      settings: AttributesFormatString=|
      | %<Table>
      | %<BreakpointsForDimension1>
      | %<BreakpointsForDimension2>
  Constant : Constant  Value=Aerodynamics.CLN_bias
      settings: AttributesFormatString=%<Value>
  Gain : Gain  Gain=Aerodynamics.CLN_scale
      settings: AttributesFormatString=%<Gain>
  Gain2 : Gain  Gain=Aerodynamics.CLN_r
      settings: AttributesFormatString=%<Gain>
  Sum1 : Sum  Inputs=+++++
  Sum2 : Sum
  Sum3 : Sum  Inputs=|++
  alpha_deg D1 : InportShadow
  alpha_deg D2 : InportShadow
  beta_deg D1 : InportShadow  Port=2
  CLN : Outport
  wires:
  r_ND_rps/1 -> Gain2/1
  Sum3/1 -> CLN/1  "CLN_B"
  beta_deg/1 -> 1-D Lookup Table1/1
  1-D Lookup Table/1 -> Sum2/1
  2-D Lookup Table2/1 -> Sum1/4  "CLN_delr"
  Sum2/1 -> Sum1/1  "CLN_0"
  alpha_deg D1/1 -> 2-D Lookup Table/1
  beta_deg D1/1 -> 2-D Lookup Table2/1
  dele_deg/1 -> 2-D Lookup Table/2
  alpha_deg D2/1 -> 2-D Lookup Table1/1
  2-D Lookup Table1/1 -> Sum1/3  "CLN_dela"
  alpha_deg/1 -> 1-D Lookup Table/1
  dela_deg/1 -> 2-D Lookup Table1/2
  Gain2/1 -> Sum1/5
  1-D Lookup Table1/1 -> Sum2/2
  delr_deg/1 -> 2-D Lookup Table2/2
  2-D Lookup Table/1 -> Sum1/2  "CLN_dele"
  Sum1/1 -> Gain/1
  Constant/1 -> Sum3/2
  Gain/1 -> Sum3/1

== system Mainframe/Non-linear Flight Dynamic Model/Subsystem1/GRM_Airframe/aerodynamics/aerodynamic_via_lookup/calc_aero_coefficients/CX_TLU ==
  alpha_deg : Inport
  beta_deg : Inport  Port=2
  dele_deg : Inport  Port=3
  dela_deg : Inport  Port=4
  delr_deg : Inport  Port=5
  2-D Lookup Table : Lookup_n-D  BreakpointsForDimension1=Aerodynamics.alpha_beta_bkpts_ind1  BreakpointsForDimension2=Aerodynamics.alpha_beta_bkpts_ind2  Table=Aerodynamics.CX_alpha_beta  ExtrapMethod=Clip  UseLastTableValue=on  InternalRulePriority=Speed  RndMeth=Simplest  InputSameDT=on
      settings: InputPortMap=u0,u1
      settings: AttributesFormatString=|
      | %<Table>
      | %<BreakpointsForDimension1>
      | %<BreakpointsForDimension2>
  2-D Lookup Table1 : Lookup_n-D  BreakpointsForDimension1=Aerodynamics.dele_inc_bkpts_ind1  BreakpointsForDimension2=Aerodynamics.dele_inc_bkpts_ind2  Table=Aerodynamics.CX_dele_inc  ExtrapMethod=Clip  UseLastTableValue=on  InternalRulePriority=Speed  RndMeth=Simplest  InputSameDT=on
      settings: InputPortMap=u0,u1
      settings: AttributesFormatString=|
      | %<Table>
      | %<BreakpointsForDimension1>
      | %<BreakpointsForDimension2>
  2-D Lookup Table2 : Lookup_n-D  BreakpointsForDimension1=Aerodynamics.dela_inc_bkpts_ind1  BreakpointsForDimension2=Aerodynamics.dela_inc_bkpts_ind2  Table=Aerodynamics.CX_dela_inc  ExtrapMethod=Clip  UseLastTableValue=on  InternalRulePriority=Speed  RndMeth=Simplest  InputSameDT=on
      settings: InputPortMap=u0,u1
      settings: AttributesFormatString=|
      | %<Table>
      | %<BreakpointsForDimension1>
      | %<BreakpointsForDimension2>
  2-D Lookup Table3 : Lookup_n-D  BreakpointsForDimension1=Aerodynamics.delr_inc_bkpts_ind1  BreakpointsForDimension2=Aerodynamics.delr_inc_bkpts_ind2  Table=Aerodynamics.CX_delr_inc  ExtrapMethod=Clip  UseLastTableValue=on  InternalRulePriority=Speed  RndMeth=Simplest  InputSameDT=on
      settings: InputPortMap=u0,u1
      settings: AttributesFormatString=|
      | %<Table>
      | %<BreakpointsForDimension1>
      | %<BreakpointsForDimension2>
  Constant : Constant  Value=Aerodynamics.CX_bias
      settings: AttributesFormatString=%<Value>
  Gain : Gain  Gain=Aerodynamics.CX_scale
      settings: AttributesFormatString=%<Gain>
  Sum : Sum  Inputs=++++
  Sum1 : Sum  Inputs=|++
  alpha_deg D1 : InportShadow
  alpha_deg D2 : InportShadow
  beta_deg D1 : InportShadow  Port=2
  CX : Outport
  wires:
  Sum/1 -> Gain/1
  2-D Lookup Table1/1 -> Sum/2  "CX_dele"
  2-D Lookup Table2/1 -> Sum/3  "CX_dela"
  2-D Lookup Table/1 -> Sum/1  "CX_0"
  alpha_deg/1 -> 2-D Lookup Table/1
  beta_deg/1 -> 2-D Lookup Table/2
  alpha_deg D1/1 -> 2-D Lookup Table1/1
  dele_deg/1 -> 2-D Lookup Table1/2
  dela_deg/1 -> 2-D Lookup Table2/2
  2-D Lookup Table3/1 -> Sum/4  "CX_delr"
  delr_deg/1 -> 2-D Lookup Table3/2
  alpha_deg D2/1 -> 2-D Lookup Table2/1
  beta_deg D1/1 -> 2-D Lookup Table3/1
  Constant/1 -> Sum1/2
  Gain/1 -> Sum1/1
  Sum1/1 -> CX/1  "CX_B"

== system Mainframe/Non-linear Flight Dynamic Model/Subsystem1/GRM_Airframe/aerodynamics/aerodynamic_via_lookup/calc_aero_coefficients/CY_TLU ==
  alpha_deg : Inport
  beta_deg : Inport  Port=2
  dele_deg : Inport  Port=3
  dela_deg : Inport  Port=4
  delr_deg : Inport  Port=5
  1-D Lookup Table : Lookup_n-D  NumberOfTableDimensions=1  BreakpointsForDimension1=Aerodynamics.alpha_bkpts_ind1  Table=Aerodynamics.CY_alpha  ExtrapMethod=Clip  UseLastTableValue=on  InternalRulePriority=Speed  RndMeth=Simplest  InputSameDT=on
      settings: AttributesFormatString=|
      | %<Table>
      | %<BreakpointsForDimension1>
  1-D Lookup Table1 : Lookup_n-D  NumberOfTableDimensions=1  BreakpointsForDimension1=Aerodynamics.beta_bkpts_ind1  Table=Aerodynamics.CY_beta  ExtrapMethod=Clip  UseLastTableValue=on  InternalRulePriority=Speed  RndMeth=Simplest  InputSameDT=on
      settings: AttributesFormatString=|
      | %<Table>
      | %<BreakpointsForDimension1>
  2-D Lookup Table : Lookup_n-D  BreakpointsForDimension1=Aerodynamics.dele_inc_bkpts_ind1  BreakpointsForDimension2=Aerodynamics.dele_inc_bkpts_ind2  Table=Aerodynamics.CY_dele_inc  ExtrapMethod=Clip  UseLastTableValue=on  InternalRulePriority=Speed  RndMeth=Simplest  InputSameDT=on
      settings: InputPortMap=u0,u1
      settings: AttributesFormatString=|
      | %<Table>
      | %<BreakpointsForDimension1>
      | %<BreakpointsForDimension2>
  2-D Lookup Table1 : Lookup_n-D  BreakpointsForDimension1=Aerodynamics.dela_inc_bkpts_ind1  BreakpointsForDimension2=Aerodynamics.dela_inc_bkpts_ind2  Table=Aerodynamics.CY_dela_inc  ExtrapMethod=Clip  UseLastTableValue=on  InternalRulePriority=Speed  RndMeth=Simplest  InputSameDT=on
      settings: InputPortMap=u0,u1
      settings: AttributesFormatString=|
      | %<Table>
      | %<BreakpointsForDimension1>
      | %<BreakpointsForDimension2>
  2-D Lookup Table2 : Lookup_n-D  BreakpointsForDimension1=Aerodynamics.delr_inc_bkpts_ind1  BreakpointsForDimension2=Aerodynamics.delr_inc_bkpts_ind2  Table=Aerodynamics.CY_delr_inc  ExtrapMethod=Clip  UseLastTableValue=on  InternalRulePriority=Speed  RndMeth=Simplest  InputSameDT=on
      settings: InputPortMap=u0,u1
      settings: AttributesFormatString=|
      | %<Table>
      | %<BreakpointsForDimension1>
      | %<BreakpointsForDimension2>
  Constant : Constant  Value=Aerodynamics.CY_bias
      settings: AttributesFormatString=%<Value>
  Gain : Gain  Gain=Aerodynamics.CY_scale
      settings: AttributesFormatString=%<Gain>
  Sum : Sum  Inputs=++++
  Sum1 : Sum
  Sum2 : Sum  Inputs=|++
  alpha_deg D1 : InportShadow
  alpha_deg D2 : InportShadow
  beta_deg D1 : InportShadow  Port=2
  CY : Outport
  wires:
  Sum2/1 -> CY/1  "CY_B"
  beta_deg/1 -> 1-D Lookup Table1/1
  1-D Lookup Table/1 -> Sum1/1
  1-D Lookup Table1/1 -> Sum1/2
  alpha_deg/1 -> 1-D Lookup Table/1
  alpha_deg D1/1 -> 2-D Lookup Table/1
  alpha_deg D2/1 -> 2-D Lookup Table1/1
  2-D Lookup Table2/1 -> Sum/4  "CY_delr"
  delr_deg/1 -> 2-D Lookup Table2/2
  2-D Lookup Table1/1 -> Sum/3  "CY_dela"
  2-D Lookup Table/1 -> Sum/2  "CY_dele"
  beta_deg D1/1 -> 2-D Lookup Table2/1
  dela_deg/1 -> 2-D Lookup Table1/2
  dele_deg/1 -> 2-D Lookup Table/2
  Sum1/1 -> Sum/1  "CY_0"
  Gain/1 -> Sum2/1
  Constant/1 -> Sum2/2
  Sum/1 -> Gain/1

== system Mainframe/Non-linear Flight Dynamic Model/Subsystem1/GRM_Airframe/aerodynamics/aerodynamic_via_lookup/calc_aero_coefficients/CZ_TLU ==
  alpha_deg : Inport
  beta_deg : Inport  Port=2
  dele_deg : Inport  Port=3
  dela_deg : Inport  Port=4
  delr_deg : Inport  Port=5
  1-D Lookup Table : Lookup_n-D  NumberOfTableDimensions=1  BreakpointsForDimension1=Aerodynamics.alpha_bkpts_ind1  Table=Aerodynamics.CZ_alpha  ExtrapMethod=Clip  UseLastTableValue=on  InternalRulePriority=Speed  RndMeth=Simplest  InputSameDT=on
      settings: AttributesFormatString=|
      | %<Table>
      | %<BreakpointsForDimension1>
  1-D Lookup Table1 : Lookup_n-D  NumberOfTableDimensions=1  BreakpointsForDimension1=Aerodynamics.beta_bkpts_ind1  Table=Aerodynamics.CZ_beta  ExtrapMethod=Clip  UseLastTableValue=on  InternalRulePriority=Speed  RndMeth=Simplest  InputSameDT=on
      settings: AttributesFormatString=|
      | %<Table>
      | %<BreakpointsForDimension1>
  2-D Lookup Table : Lookup_n-D  BreakpointsForDimension1=Aerodynamics.dele_inc_bkpts_ind1  BreakpointsForDimension2=Aerodynamics.dele_inc_bkpts_ind2  Table=Aerodynamics.CZ_dele_inc  ExtrapMethod=Clip  UseLastTableValue=on  InternalRulePriority=Speed  RndMeth=Simplest  InputSameDT=on
      settings: InputPortMap=u0,u1
      settings: AttributesFormatString=|
      | %<Table>
      | %<BreakpointsForDimension1>
      | %<BreakpointsForDimension2>
  2-D Lookup Table1 : Lookup_n-D  BreakpointsForDimension1=Aerodynamics.dela_inc_bkpts_ind1  BreakpointsForDimension2=Aerodynamics.dela_inc_bkpts_ind2  Table=Aerodynamics.CZ_dela_inc  ExtrapMethod=Clip  UseLastTableValue=on  InternalRulePriority=Speed  RndMeth=Simplest  InputSameDT=on
      settings: InputPortMap=u0,u1
      settings: AttributesFormatString=|
      | %<Table>
      | %<BreakpointsForDimension1>
      | %<BreakpointsForDimension2>
  2-D Lookup Table2 : Lookup_n-D  BreakpointsForDimension1=Aerodynamics.delr_inc_bkpts_ind1  BreakpointsForDimension2=Aerodynamics.delr_inc_bkpts_ind2  Table=Aerodynamics.CZ_delr_inc  ExtrapMethod=Clip  UseLastTableValue=on  InternalRulePriority=Speed  RndMeth=Simplest  InputSameDT=on
      settings: InputPortMap=u0,u1
      settings: AttributesFormatString=|
      | %<Table>
      | %<BreakpointsForDimension1>
      | %<BreakpointsForDimension2>
  Constant : Constant  Value=Aerodynamics.CZ_bias
      settings: AttributesFormatString=%<Value>
  Gain : Gain  Gain=Aerodynamics.CZ_scale
      settings: AttributesFormatString=%<Gain>
  Sum : Sum  Inputs=++++
  Sum1 : Sum
  Sum2 : Sum  Inputs=|++
  alpha_deg D1 : InportShadow
  alpha_deg D2 : InportShadow
  beta_deg D1 : InportShadow  Port=2
  CZ : Outport
  wires:
  dele_deg/1 -> 2-D Lookup Table/2
  dela_deg/1 -> 2-D Lookup Table1/2
  beta_deg D1/1 -> 2-D Lookup Table2/1
  2-D Lookup Table/1 -> Sum/2  "CZ_dele"
  2-D Lookup Table1/1 -> Sum/3  "CZ_dela"
  delr_deg/1 -> 2-D Lookup Table2/2
  2-D Lookup Table2/1 -> Sum/4  "CZ_delr"
  alpha_deg D2/1 -> 2-D Lookup Table1/1
  alpha_deg D1/1 -> 2-D Lookup Table/1
  alpha_deg/1 -> 1-D Lookup Table/1
  1-D Lookup Table1/1 -> Sum1/2
  1-D Lookup Table/1 -> Sum1/1
  Sum1/1 -> Sum/1  "CZ_0"
  beta_deg/1 -> 1-D Lookup Table1/1
  Sum2/1 -> CZ/1  "CZ_B"
  Constant/1 -> Sum2/2
  Gain/1 -> Sum2/1
  Sum/1 -> Gain/1

== system Mainframe/Non-linear Flight Dynamic Model/Subsystem1/GRM_Airframe/aerodynamics/aerodynamic_via_lookup/calc_aero_for_mom/create_pAPB ==
  Constant : Constant  Value=Aerodynamics.xcg
      settings: AttributesFormatString=%<Value>
  Constant3 : Constant  Value=0
  Gain : Gain  Gain=-1
  Vector Concatenate : Concatenate  NumInputs=3
  pAPB : Outport  VectorParamsAs1DForOutWhenUnconnected=off
  wires:
  Constant3/1 -> Vector Concatenate/3, Vector Concatenate/2
  Gain/1 -> Vector Concatenate/1
  Constant/1 -> Gain/1
  Vector Concatenate/1 -> pAPB/1  "pAPB"

== system Mainframe/Non-linear Flight Dynamic Model/Subsystem1/GRM_Airframe/aerodynamics/aerodynamic_via_lookup/calc_aero_for_mom/cross_product ==
  note: Outputs [size]:
      |
      | r1 x r2  [3x1]
  note: Inputs [size]:
      |
      | r1 [3x1]
      | r2 [3x1]
  r1 : Inport
  r2 : Inport  Port=2
  Demux2 : Demux  Outputs=[1;1;1]
      settings: DisplayOption=none
  Demux3 : Demux  Outputs=[1;1;1]
      settings: DisplayOption=none
  Product{2..7} (6 alike) : Product  InputSameDT=on  RndMeth=Zero  SaturateOnIntegerOverflow=on  OutDataTypeStr=Inherit: Same as first input
  Sum : Sum  Inputs=+-  InputSameDT=on  SaturateOnIntegerOverflow=on  OutDataTypeStr=Inherit: Same as first input
  Sum1 : Sum  Inputs=+-  InputSameDT=on  SaturateOnIntegerOverflow=on  OutDataTypeStr=Inherit: Same as first input
  Sum2 : Sum  Inputs=+-  InputSameDT=on  SaturateOnIntegerOverflow=on  OutDataTypeStr=Inherit: Same as first input
  Vector Concatenate : Concatenate  NumInputs=3
  r1_x_r2 : Outport  PortDimensions=[3,1]  VectorParamsAs1DForOutWhenUnconnected=off
  wires:
  Demux2/2 -> Product2/1, Product7/1
  Demux3/3 -> Product5/2, Product2/2
  Demux3/2 -> Product6/2, Product3/2
  Demux2/3 -> Product3/1, Product4/1
  Demux3/1 -> Product7/2, Product4/2
  Demux2/1 -> Product6/1, Product5/1
  Product2/1 -> Sum/1
  Product3/1 -> Sum/2
  Product4/1 -> Sum1/1
  Product5/1 -> Sum1/2
  Product6/1 -> Sum2/1
  Product7/1 -> Sum2/2
  Sum/1 -> Vector Concatenate/1
  Sum1/1 -> Vector Concatenate/2
  Sum2/1 -> Vector Concatenate/3
  r1/1 -> Demux2/1
  r2/1 -> Demux3/1
  Vector Concatenate/1 -> r1_x_r2/1

== system Mainframe/Non-linear Flight Dynamic Model/Subsystem1/GRM_Airframe/aerodynamics/aerodynamic_via_lookup/calc_aero_for_mom/launch_rail ==
  hBE : Inport
  FBAB_c : Inport  Port=2
  Constant1 : Constant  Value=flag_I_aero_switch
  Constant3 : Constant  Value=0
  Subtract : Sum  Inputs=++-
  Switch : Switch  Criteria=u2 > Threshold  Threshold=0.05
  Vector Concatenate : Concatenate  NumInputs=3
  initial_altitude : Subsystem
  FBAB : Outport  VectorParamsAs1DForOutWhenUnconnected=off
  wires:
  Constant1/1 -> Subtract/2
  hBE/1 -> Subtract/1
  Subtract/1 -> Switch/2
  Constant3/1 -> Vector Concatenate/1, Vector Concatenate/2, Vector Concatenate/3
  Switch/1 -> FBAB/1  "FBAB"
  Vector Concatenate/1 -> Switch/3
  FBAB_c/1 -> Switch/1
  initial_altitude/1(hBE_0) -> Subtract/3

== system Mainframe/Non-linear Flight Dynamic Model/Subsystem1/GRM_Airframe/aerodynamics/aerodynamic_via_lookup/calc_aero_for_mom/launch_rail1 ==
  hBE : Inport
  MBAB_c : Inport  Port=2
  Constant1 : Constant  Value=flag_I_aero_switch
  Constant3 : Constant  Value=0
  Subtract : Sum  Inputs=++-
  Switch : Switch  Criteria=u2 > Threshold  Threshold=0.05
  Vector Concatenate : Concatenate  NumInputs=3
  initial_altitude : Subsystem
  MBAB : Outport  VectorParamsAs1DForOutWhenUnconnected=off
  wires:
  initial_altitude/1(hBE_0) -> Subtract/3
  MBAB_c/1 -> Switch/1
  Vector Concatenate/1 -> Switch/3
  Switch/1 -> MBAB/1  "MBAB"
  Constant3/1 -> Vector Concatenate/3, Vector Concatenate/2, Vector Concatenate/1
  Subtract/1 -> Switch/2
  hBE/1 -> Subtract/1
  Constant1/1 -> Subtract/2

== system Mainframe/Non-linear Flight Dynamic Model/Subsystem1/GRM_Airframe/environment/WGS84_Gravitation/WGS84_2_ECEF/WGS84 Transformation Parameter  ==
  phi : Inport
  Add2 : Sum  Inputs=+-
  Divide : Product  Inputs=**
  Divide1 : Product  Inputs=**
  Divide2 : Product  Inputs=**
  Divide3 : Product  Inputs=/*
  Sqrt : Sqrt  SaturateOnIntegerOverflow=on
  Subsystem : Subsystem
  Trigonometric Function : Trigonometry
  "WGS84 Semi-major Axis, [m]" : Constant  Value=c_rsma
  "WGS84 Semi-minor Axis, [m]" : Constant  Value=c_b_WGS
  a3 : Constant
  N : Outport  VectorParamsAs1DForOutWhenUnconnected=off
  e : Outport  Port=2  VectorParamsAs1DForOutWhenUnconnected=off
  wires:
  "WGS84 Semi-minor Axis, [m]"/1 -> Subsystem/1(b)  "c_b_WGS"
  "WGS84 Semi-major Axis, [m]"/1 -> Subsystem/2(a), Divide3/2  "c_rsma"
  Divide1/1 -> Divide2/1  "sin(phi)^2"
  Divide3/1 -> N/1  "N"
  Sqrt/1 -> Divide3/1
  a3/1 -> Add2/1
  Divide2/1 -> Add2/2
  Trigonometric Function/1 -> Divide1/2, Divide1/1
  Divide/1 -> Divide2/2  "e^2"
  Subsystem/1(e) -> e/1, Divide/2, Divide/1
  Add2/1 -> Sqrt/1
  phi/1 -> Trigonometric Function/1

== system Mainframe/Non-linear Flight Dynamic Model/Subsystem1/GRM_Airframe/environment/atmosphere_static_ISO_2533/tmp_and_pressure_ISO_2533/static_Temperature ==
  Tmp_ref : Inport
  h_geop : Inport  Port=2
  h_geop_ref : Inport  Port=3
  Add : Sum
  Product : Product
  Subtract : Sum  Inputs=+-
  Tmp_gradient_tropo : Constant  Value=c_be
  Tmp : Outport  VectorParamsAs1DForOutWhenUnconnected=off
  wires:
  Subtract/1 -> Product/2
  Tmp_gradient_tropo/1 -> Product/1
  Product/1 -> Add/2
  Add/1 -> Tmp/1  "Tmp"
  Tmp_ref/1 -> Add/1
  h_geop/1 -> Subtract/1
  h_geop_ref/1 -> Subtract/2
